simulink model "zeros_step_response_model"  (R2021a)
settings: Solver=VariableStepAuto  StartTime=0.0  StopTime=10.0  RelTol=1e-3
values from neighbouring files (symbols this model uses):
  B = 20000    [lab2.m]
  J = 600000    [lab2.m]
settings Model: Creator=LEGION  LastModifiedBy=LEGION

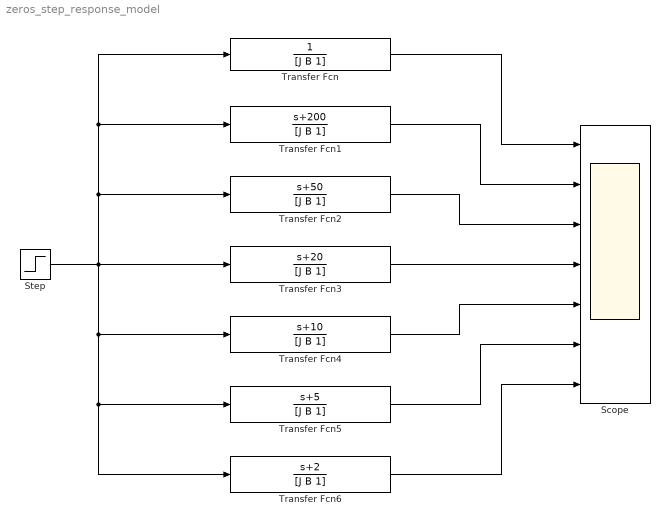
== system zeros_step_response_model ==
  Scope : Scope  NumInputPorts=7
  Step : Step  SampleTime=0
  Transfer Fcn : TransferFcn  Denominator=[J B 1]
  Transfer Fcn1 : TransferFcn  Numerator=[1 200]  Denominator=[J B 1]
  Transfer Fcn2 : TransferFcn  Numerator=[1 50]  Denominator=[J B 1]
  Transfer Fcn3 : TransferFcn  Numerator=[1 20]  Denominator=[J B 1]
  Transfer Fcn4 : TransferFcn  Numerator=[1 10]  Denominator=[J B 1]
  Transfer Fcn5 : TransferFcn  Numerator=[1 5]  Denominator=[J B 1]
  Transfer Fcn6 : TransferFcn  Numerator=[1 2]  Denominator=[J B 1]
  wires:
  Transfer Fcn1/1 -> Scope/2
  Transfer Fcn2/1 -> Scope/3
  Transfer Fcn4/1 -> Scope/5
  Transfer Fcn/1 -> Scope/1
  Transfer Fcn3/1 -> Scope/4
  Step/1 -> Transfer Fcn2/1, Transfer Fcn1/1, Transfer Fcn/1, Transfer Fcn6/1, Transfer Fcn5/1, Transfer Fcn4/1, Transfer Fcn3/1
  Transfer Fcn5/1 -> Scope/6
  Transfer Fcn6/1 -> Scope/7
